simulink model "SchemaControlloDecentralizzatoSmartSixR2013a"  (Simulink 8.7)
settings: Solver=ode45  StartTime=0.0  StopTime=t(end)+Tf  FixedStep=T  MaxStep=T  RelTol=1e-3
PreLoadFcn:
  | initFunction
InitFcn:
  | initFunction
StopFcn:
  | cd ..
  | 
  | figure
  | subplot(31,1)
  | plot(err_q.data(1:50))
  | subplot(312)
  | plot(err_dq.data(1:50))
  | subplot(313)
  | plot(err_ddq.data(1:50))
values from neighbouring files (symbols this model uses):
  FM = Kr^-1*Fv*Kr^-1    [initFunction.m]
  Im = Kr^-1*Bconst*Kr^-1    [initFunction.m]
  KCA = [586.881582263 0 0 0 0 0 0 566.981582263 0 0 0 0 ... (36 elements, 6x6)]    [KCA.mat]
  KCP = [63 0 0 0 0 0 0 63 0 0 0 0 ... (36 elements, 6x6)]    [KCP.mat]
  KCV = [315.577034284 0 0 0 0 0 0 325.715347644 0 0 0 0 ... (36 elements, 6x6)]    [KCV.mat]    (also in initFunction.m = KCV*rKCV^-1)
  KM = [0.0232558139535 0 0 0 0 0 0 0.0158982511924 0 0 0 0 ... (36 elements, 6x6)]    [KM.mat]
  Kr = diag(kr)    [ParametriMotori.m]
  Kt = diag(kt)    [ParametriMotori.m]
  KTA = [1 0 0 0 0 0 0 1 0 0 0 0 ... (36 elements, 6x6)]    [KTA.mat]
  KTP = [1 0 0 0 0 0 0 1 0 0 0 0 ... (36 elements, 6x6)]    [KTP.mat]
  KTV = [1 0 0 0 0 0 0 1 0 0 0 0 ... (36 elements, 6x6)]    [KTV.mat]
  Kv = diag(kv)    [ParametriMotori.m]
  La = diag(la)    [ParametriMotori.m]
  q0 = q0'    [initFunction.m]
  Ra = diag(ra)    [ParametriMotori.m]
  T = Tf    (= 0.002)    [initFunction.m]
  TCA = [4.96122857983e-05 0 0 0 0 0 0 3.97711481373e-05 0 0 0 0 ... (36 elements, 6x6)]    [TCA.mat]
libraries: simulink x18
(part 1 of 2)
CloseFcn:
  | rtwprivate ssgencode ModelCloseRequest ContributiCoppieComau
settings Model: Creator=Alessandro  LastModifiedBy=Gianluigi  ExtModeAutoUpdateStatusClock=off
settings DataIOCC: SaveFormat=StructureWithTime
settings OptimizationCC: BlockReduction=off  BufferReuse=off  ExpressionDepthLimit=2147483647  InitFltsAndDblsToZero=on
settings DebuggingCC: AlgebraicLoopMsg=none  SaveWithParameterizedLinksMsg=none  SignalResolutionControl=TryResolveAllWithWarning  InheritedTsInSrcMsg=none  MultiTaskDSMMsg=warning  MultiTaskCondExecSysMsg=none  TasksWithSamePriorityMsg=none  FcnCallInpInsideContextMsg=UseLocalSettings  UnconnectedInputMsg=none  UnconnectedOutputMsg=none  UnconnectedLineMsg=none  StateNameClashWarn=warning
settings GRTTargetCC: TargetFcnLib=ansi_tfl_tmw.mat  CombineOutputUpdateFcns=off  GRTInterface=on

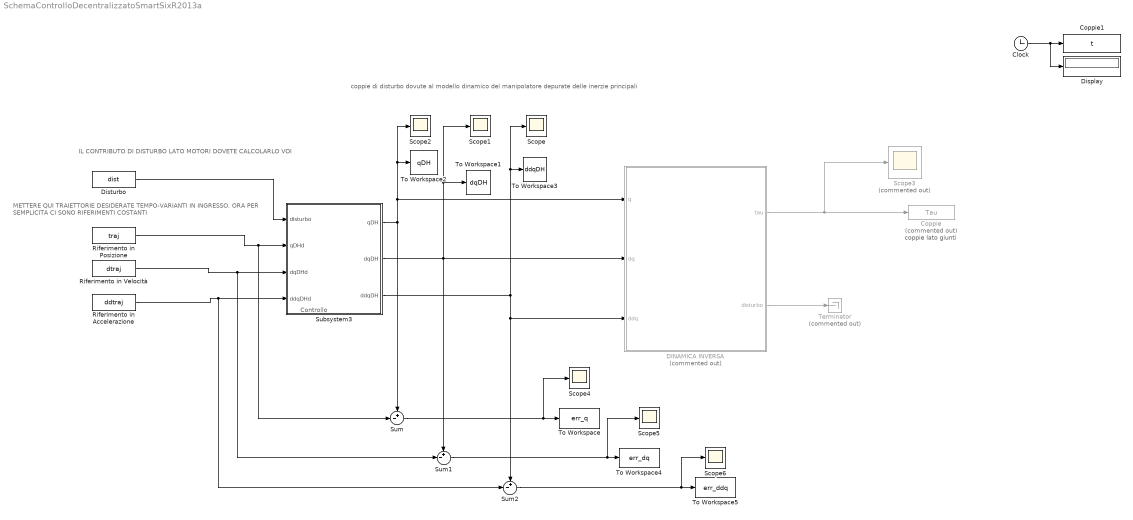
== system SchemaControlloDecentralizzatoSmartSixR2013a ==
  note: coppie di disturbo dovute al modello dinamico del manipolatore depurate delle inerzie principali
  note: Controllo
  note: METTERE QUI TRAIETTORIE DESIDERATE TEMPO-VARIANTI IN INGRESSO.
      | ORA PER SEMPLICITA CI SONO RIFERIMENTI COSTANTI
  note: coppie lato giunti
  note: IL CONTRIBUTO DI DISTURBO LATO MOTORI DOVETE CALCOLARLO VOI
  Clock : Clock
  Coppie : ToWorkspace  Commented=on  VariableName=Tau  SampleTime=-1
  Coppie1 : ToWorkspace  VariableName=t  SampleTime=-1
  DINAMICA INVERSA : Subsystem  Commented=on
      mask Display:
      | disp('Contributi Coppie');
      | port_label('input', 1, 'qDH');
      | port_label('input', 2, 'dqDH');
      | port_label('input', 3, 'ddqDH');
      | port_label('output', 1, 'Coppie Complessive');
      | port_label('output', 2, 'Disturbo lato motori');
  Display : Display
  Disturbo : FromWorkspace  VariableName=dist  Interpolate=off  OutputAfterFinalValue=Holding final value
  Riferimento in Accelerazione : FromWorkspace  VariableName=ddtraj  OutputAfterFinalValue=Holding final value
  Riferimento in Posizione : FromWorkspace  VariableName=traj  Interpolate=off  OutputAfterFinalValue=Holding final value
  Riferimento in Velocità : FromWorkspace  VariableName=dtraj  Interpolate=off  OutputAfterFinalValue=Holding final value
  Scope{,1..2,4..6} (6 alike) : Scope
  Scope3 : Scope  Commented=on
  Subsystem3 : Subsystem
      mask Display:
      | disp('Controllo');
      | port_label('input', 1, 'disturbo');
      | port_label('input', 2, 'qDHd');
      | port_label('input', 3, 'dqDHd');
      | port_label('output', 1, 'qDH');
      | port_label('output', 2, 'dqDH');
      | port_label('output', 3, 'ddqDH');
  Sum : Sum  Inputs=+-|
  Sum1 : Sum  Inputs=+-|
  Sum2 : Sum  Inputs=+-|
  Terminator : Terminator  Commented=on
  To Workspace : ToWorkspace  VariableName=err_q  SaveFormat=Timeseries  SampleTime=-1
  To Workspace1 : ToWorkspace  VariableName=dqDH  SampleTime=-1
  To Workspace2 : ToWorkspace  VariableName=qDH  SampleTime=-1
  To Workspace3 : ToWorkspace  VariableName=ddqDH  SampleTime=-1
  To Workspace4 : ToWorkspace  VariableName=err_dq  SaveFormat=Timeseries  SampleTime=-1
  To Workspace5 : ToWorkspace  VariableName=err_ddq  SaveFormat=Timeseries  SampleTime=-1
  wires:
  Clock/1 -> Coppie1/1, Display/1
  Subsystem3/2(dqDH) -> Sum1/1, To Workspace1/1, Scope1/1, DINAMICA INVERSA/2(dq)
  DINAMICA INVERSA/1(tau) -> Coppie/1, Scope3/1
  Subsystem3/1(qDH) -> DINAMICA INVERSA/1(q), To Workspace2/1, Scope2/1, Sum/1
  Subsystem3/3(ddqDH) -> Sum2/1, DINAMICA INVERSA/3(ddq), To Workspace3/1, Scope/1
  Riferimento in Velocità/1 -> Sum1/2, Subsystem3/3(dqDHd)
  Riferimento in Accelerazione/1 -> Sum2/2, Subsystem3/4(ddqDHd)
  Riferimento in Posizione/1 -> Sum/2, Subsystem3/2(qDHd)
  Disturbo/1 -> Subsystem3/1(disturbo)
  DINAMICA INVERSA/2(disturbo) -> Terminator/1
  Sum/1 -> Scope4/1, To Workspace/1
  Sum1/1 -> Scope5/1, To Workspace4/1
  Sum2/1 -> Scope6/1, To Workspace5/1

== system SchemaControlloDecentralizzatoSmartSixR2013a/DINAMICA INVERSA ==
  note: IL CONTRIBUTO DI DISTURBO LATO MOTORI DOVETE CALCOLARLO VOI
  q : Inport
  dq : Inport  Port=2
  ddq : Inport  Port=3
  Add : Sum  Inputs=++++
  Constant : Constant  Value=[1 1 1 1 1 1]
  Demux : Demux
  Dinamica Inversa : MATLABFcn  MATLABFcn=CalcCoppieComau  OutputDimensions=24
  Mux : Mux  Inputs=3
  To Workspace1 : ToWorkspace  VariableName=tauCentrifugo  SampleTime=-1
  To Workspace2 : ToWorkspace  VariableName=tauAttrViscoso  SampleTime=-1
  To Workspace4 : ToWorkspace  VariableName=tauInerzia  SampleTime=-1
  To Workspace5 : ToWorkspace  VariableName=tauGravita  SampleTime=-1
  tau : Outport
  disturbo : Outport  Port=2
  wires:
  q/1 -> Mux/1
  Mux/1 -> Dinamica Inversa/1
  dq/1 -> Mux/2
  ddq/1 -> Mux/3
  Dinamica Inversa/1 -> Demux/1
  Add/1 -> tau/1
  Demux/1 -> Add/1, To Workspace4/1
  Demux/2 -> Add/2, To Workspace1/1
  Demux/3 -> Add/3, To Workspace2/1
  Demux/4 -> Add/4, To Workspace5/1
  Constant/1 -> disturbo/1

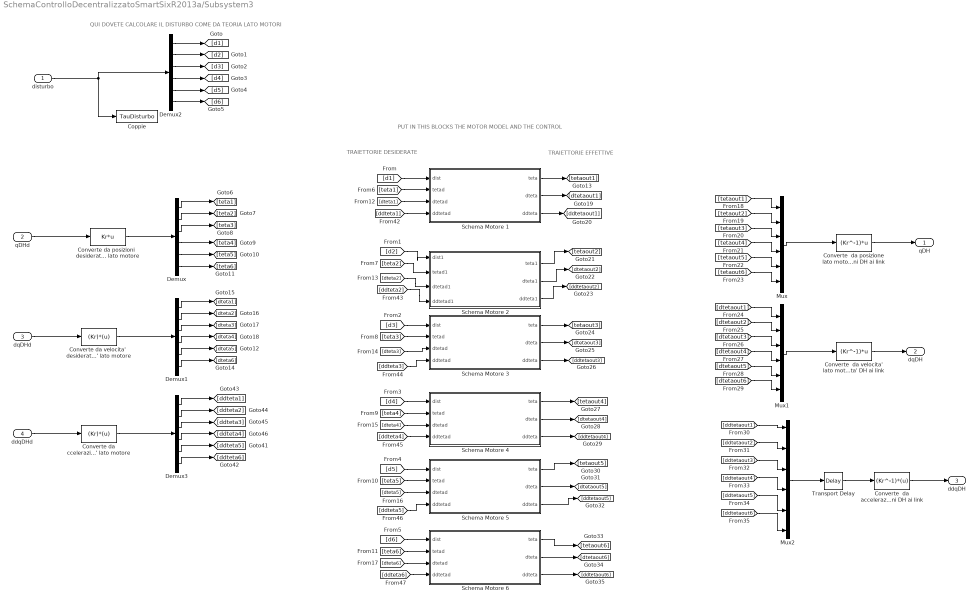
== system SchemaControlloDecentralizzatoSmartSixR2013a/Subsystem3 ==
  note: PUT IN THIS BLOCKS THE MOTOR MODEL AND THE CONTROL
  note: TRAIETTORIE DESIDERATE
  note: TRAIETTORIE EFFETTIVE
  note: QUI DOVETE CALCOLARE IL DISTURBO COME DA TEORIA LATO MOTORI
  disturbo : Inport
  qDHd : Inport  Port=2
  dqDHd : Inport  Port=3
  ddqDHd : Inport  Port=4
  Converte  da accelerazioni lato motore  ad accelerazioni DH ai link : MATLABFcn  MATLABFcn=(Kr^-1)*(u)
  "Converte  da posizione lato motore a  posizioni DH ai link " : MATLABFcn  MATLABFcn=(Kr^-1)*u
  "Converte  da velocita' lato motore  a velocita' DH ai link " : MATLABFcn  MATLABFcn=(Kr^-1)*u
  Converte da ccelerazioni  desiderate DH ai link  in velocita' lato motore : MATLABFcn  MATLABFcn=(Kr)*(u)
  "Converte da posizioni  desiderate DH ai link  in posizione lato motore " : MATLABFcn  MATLABFcn=Kr*u
  "Converte da velocita'  desiderate DH ai link  in velocita' lato motore " : MATLABFcn  MATLABFcn=(Kr)*(u)
  Coppie : ToWorkspace  VariableName=TauDisturbo  SampleTime=-1
  Demux{,1..3} (4 alike) : Demux  Outputs=6
  Mux : Mux  Inputs=6
  Mux1 : Mux  Inputs=6
  Mux2 : Mux  Inputs=6
  Schema Motore 1 : Subsystem  mask{i=1}
  Schema Motore 2 : Subsystem  mask{i=2}
  Schema Motore 3 : Subsystem  mask{i=3}
  Schema Motore 4 : Subsystem  mask{i=4}
  Schema Motore 5 : Subsystem  mask{i=5}
  Schema Motore 6 : Subsystem  mask{i=6}
  Transport Delay : TransportDelay  DelayTime=T
  qDH : Outport
  dqDH : Outport  Port=2
  ddqDH : Outport  Port=3
  wires:
  qDHd/1 -> "Converte da posizioni  desiderate DH ai link  in posizione lato motore "/1
  dqDHd/1 -> "Converte da velocita'  desiderate DH ai link  in velocita' lato motore "/1
  "Converte  da velocita' lato motore  a velocita' DH ai link "/1 -> dqDH/1
  Converte  da accelerazioni lato motore  ad accelerazioni DH ai link/1 -> ddqDH/1
  "Converte da posizioni  desiderate DH ai link  in posizione lato motore "/1 -> Demux/1
  disturbo/1 -> Coppie/1, Demux2/1
  "Converte  da posizione lato motore a  posizioni DH ai link "/1 -> qDH/1
  Mux/1 -> "Converte  da posizione lato motore a  posizioni DH ai link "/1
  Demux2/1 -> [d1]
  Demux2/2 -> [d2]
  Demux2/3 -> [d3]
  Demux2/4 -> [d4]
  Demux2/5 -> [d5]
  Demux2/6 -> [d6]
  [d3] -> Schema Motore 3/1(dist)
  [d4] -> Schema Motore 4/1(dist)
  [d5] -> Schema Motore 5/1(dist)
  [d6] -> Schema Motore 6/1(dist)
  Demux/1 -> [teta1]
  Demux/2 -> [teta2]
  Demux/3 -> [teta3]
  Demux/4 -> [teta4]
  Demux/5 -> [teta5]
  Demux/6 -> [teta6]
  [teta3] -> Schema Motore 3/2(tetad)
  [teta4] -> Schema Motore 4/2(tetad)
  [teta5] -> Schema Motore 5/2(tetad)
  [teta6] -> Schema Motore 6/2(tetad)
  "Converte da velocita'  desiderate DH ai link  in velocita' lato motore "/1 -> Demux1/1
  Demux1/1 -> [dteta1]
  Demux1/2 -> [dteta2]
  Demux1/3 -> [dteta3]
  Demux1/4 -> [dteta4]
  Demux1/5 -> [dteta5]
  Demux1/6 -> [dteta6]
  [dteta3] -> Schema Motore 3/3(dtetad)
  [dteta4] -> Schema Motore 4/3(dtetad)
  [dteta5] -> Schema Motore 5/3(dtetad)
  [dteta6] -> Schema Motore 6/3(dtetad)
  [tetaout1] -> Mux/1
  [tetaout2] -> Mux/2
  [tetaout3] -> Mux/3
  [tetaout4] -> Mux/4
  [tetaout5] -> Mux/5
  [tetaout6] -> Mux/6
  Mux1/1 -> "Converte  da velocita' lato motore  a velocita' DH ai link "/1
  [dtetaout1] -> Mux1/1
  [dtetaout2] -> Mux1/2
  [dtetaout3] -> Mux1/3
  [dtetaout4] -> Mux1/4
  [dtetaout5] -> Mux1/5
  [dtetaout6] -> Mux1/6
  [ddtetaout1] -> Mux2/1
  [ddtetaout2] -> Mux2/2
  [ddtetaout3] -> Mux2/3
  [ddtetaout4] -> Mux2/4
  [ddtetaout5] -> Mux2/5
  [ddtetaout6] -> Mux2/6
  [teta1] -> Schema Motore 1/2(tetad)
  [dteta1] -> Schema Motore 1/3(dtetad)
  Schema Motore 1/1(teta) -> [tetaout1]
  Schema Motore 1/2(dteta) -> [dtetaout1]
  Schema Motore 1/3(ddteta) -> [ddtetaout1]
  [d1] -> Schema Motore 1/1(dist)
  ddqDHd/1 -> Converte da ccelerazioni  desiderate DH ai link  in velocita' lato motore/1
  Demux3/1 -> [ddteta1]
  Demux3/2 -> [ddteta2]
  Demux3/3 -> [ddteta3]
  Demux3/4 -> [ddteta4]
  Demux3/5 -> [ddteta5]
  Demux3/6 -> [ddteta6]
  Converte da ccelerazioni  desiderate DH ai link  in velocita' lato motore/1 -> Demux3/1
  [ddteta1] -> Schema Motore 1/4(ddtetad)
  Schema Motore 3/1(teta) -> [tetaout3]
  Schema Motore 3/2(dteta) -> [dtetaout3]
  Schema Motore 3/3(ddteta) -> [ddtetaout3]
  Schema Motore 4/1(teta) -> [tetaout4]
  Schema Motore 4/2(dteta) -> [dtetaout4]
  Schema Motore 4/3(ddteta) -> [ddtetaout4]
  Schema Motore 5/1(teta) -> [tetaout5]
  Schema Motore 5/2(dteta) -> [dtetaout5]
  Schema Motore 5/3(ddteta) -> [ddtetaout5]
  Schema Motore 6/1(teta) -> [tetaout6]
  Schema Motore 6/2(dteta) -> [dtetaout6]
  Schema Motore 6/3(ddteta) -> [ddtetaout6]
  [ddteta3] -> Schema Motore 3/4(ddtetad)
  [ddteta4] -> Schema Motore 4/4(ddtetad)
  [ddteta5] -> Schema Motore 5/4(ddtetad)
  [ddteta6] -> Schema Motore 6/4(ddtetad)
  [d2] -> Schema Motore 2/1(dist1)
  [teta2] -> Schema Motore 2/2(tetad1)
  [dteta2] -> Schema Motore 2/3(dtetad1)
  [ddteta2] -> Schema Motore 2/4(ddtetad1)
  Schema Motore 2/1(teta1) -> [tetaout2]
  Schema Motore 2/2(dteta1) -> [dtetaout2]
  Schema Motore 2/3(ddteta1) -> [ddtetaout2]
  Mux2/1 -> Transport Delay/1
  Transport Delay/1 -> Converte  da accelerazioni lato motore  ad accelerazioni DH ai link/1

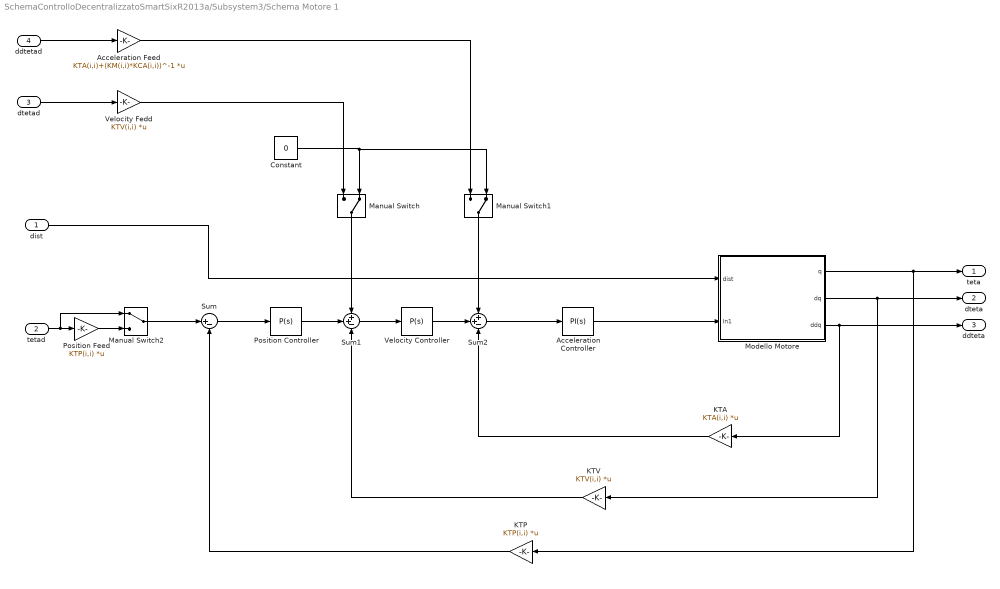
== system SchemaControlloDecentralizzatoSmartSixR2013a/Subsystem3/Schema Motore 1 ==
  dist : Inport  PortDimensions=1
  tetad : Inport  Port=2  PortDimensions=1
  dtetad : Inport  Port=3  PortDimensions=1
  ddtetad : Inport  Port=4  PortDimensions=1
  Acceleration Controller : simulink/Continuous/PID Controller  Controller=PI  TimeDomain=Continuous-time  SampleTime=-1  IntegratorMethod=Forward Euler  FilterMethod=Forward Euler  Form=Parallel  UseFilter=on  ControllerParametersSource=internal  P=TCA(i,i)*KCA(i,i)  I=KCA(i,i)  D=0  N=100  InitialConditionSource=internal  InitialConditionForIntegrator=0  InitialConditionForFilter=0  ExternalReset=none  LimitOutput=off  UpperSaturationLimit=inf  LowerSaturationLimit=-inf  LinearizeAsGain=on  AntiWindupMode=none  Kb=1  TrackingMode=off  Kt=1  PParamMin=[]  PParamMax=[]  IParamMin=[]  IParamMax=[]  DParamMin=[]  DParamMax=[]  NParamMin=[]  NParamMax=[]  KbParamMin=[]  KbParamMax=[]  KtParamMin=[]  KtParamMax=[]  POutMin=[]  POutMax=[]  IOutMin=[]  IOutMax=[]  DOutMin=[]  DOutMax=[]  NOutMin=[]  NOutMax=[]  KbOutMin=[]  KbOutMax=[]  KtOutMin=[]  KtOutMax=[]  IntegratorOutMin=[]  IntegratorOutMax=[]  FilterOutMin=[]  FilterOutMax=[]  SumOutMin=[]  SumOutMax=[]  SumI1OutMin=[]  SumI1OutMax=[]  SumI2OutMin=[]  SumI2OutMax=[]  SumI3OutMin=[]  SumI3OutMax=[]  SumDOutMin=[]  SumDOutMax=[]  SaturationOutMin=[]  SaturationOutMax=[]  IntegratorContinuousStateAttributes=''  IntegratorStateMustResolveToSignalObject=off  IntegratorRTWStateStorageClass=Auto  FilterContinuousStateAttributes=''  FilterStateMustResolveToSignalObject=off  FilterRTWStateStorageClass=Auto  DifferentiatorICPrevScaledInput=0  DifferentiatorOutMin=[]  DifferentiatorOutMax=[]
  Acceleration Feed : Gain  Gain=KTA(i,i)+(KM(i,i)*KCA(i,i))^-1  Multiplication=Matrix(K*u)
  Constant : Constant  Value=0
  KTA : Gain  Gain=KTA(i,i)  Multiplication=Matrix(K*u)
  KTP : Gain  Gain=KTP(i,i)  Multiplication=Matrix(K*u)
  KTV : Gain  Gain=KTV(i,i)  Multiplication=Matrix(K*u)
  Manual Switch : ManualSwitch  CurrentSetting=0
  Manual Switch1 : ManualSwitch  CurrentSetting=0
  Manual Switch2 : ManualSwitch
  Modello Motore : Subsystem
  Position Controller : simulink/Continuous/PID Controller  Controller=P  TimeDomain=Continuous-time  SampleTime=-1  IntegratorMethod=Forward Euler  FilterMethod=Forward Euler  Form=Parallel  UseFilter=on  ControllerParametersSource=internal  P=KCP(i,i)  I=1  D=0  N=100  InitialConditionSource=internal  InitialConditionForIntegrator=0  InitialConditionForFilter=0  ExternalReset=none  LimitOutput=off  UpperSaturationLimit=inf  LowerSaturationLimit=-inf  LinearizeAsGain=on  AntiWindupMode=none  Kb=1  TrackingMode=off  Kt=1  PParamMin=[]  PParamMax=[]  IParamMin=[]  IParamMax=[]  DParamMin=[]  DParamMax=[]  NParamMin=[]  NParamMax=[]  KbParamMin=[]  KbParamMax=[]  KtParamMin=[]  KtParamMax=[]  POutMin=[]  POutMax=[]  IOutMin=[]  IOutMax=[]  DOutMin=[]  DOutMax=[]  NOutMin=[]  NOutMax=[]  KbOutMin=[]  KbOutMax=[]  KtOutMin=[]  KtOutMax=[]  IntegratorOutMin=[]  IntegratorOutMax=[]  FilterOutMin=[]  FilterOutMax=[]  SumOutMin=[]  SumOutMax=[]  SumI1OutMin=[]  SumI1OutMax=[]  SumI2OutMin=[]  SumI2OutMax=[]  SumI3OutMin=[]  SumI3OutMax=[]  SumDOutMin=[]  SumDOutMax=[]  SaturationOutMin=[]  SaturationOutMax=[]  IntegratorContinuousStateAttributes=''  IntegratorStateMustResolveToSignalObject=off  IntegratorRTWStateStorageClass=Auto  FilterContinuousStateAttributes=''  FilterStateMustResolveToSignalObject=off  FilterRTWStateStorageClass=Auto  DifferentiatorICPrevScaledInput=0  DifferentiatorOutMin=[]  DifferentiatorOutMax=[]
  Position Feed : Gain  Gain=KTP(i,i)  Multiplication=Matrix(K*u)
  Sum : Sum  Inputs=|+-
  Sum1 : Sum  Inputs=++-
  Sum2 : Sum  Inputs=++-
  Velocity Controller : simulink/Continuous/PID Controller  Controller=P  TimeDomain=Continuous-time  SampleTime=-1  IntegratorMethod=Forward Euler  FilterMethod=Forward Euler  Form=Parallel  UseFilter=on  ControllerParametersSource=internal  P=KCV(i,i)  I=1  D=0  N=100  InitialConditionSource=internal  InitialConditionForIntegrator=0  InitialConditionForFilter=0  ExternalReset=none  LimitOutput=off  UpperSaturationLimit=inf  LowerSaturationLimit=-inf  LinearizeAsGain=on  AntiWindupMode=none  Kb=1  TrackingMode=off  Kt=1  PParamMin=[]  PParamMax=[]  IParamMin=[]  IParamMax=[]  DParamMin=[]  DParamMax=[]  NParamMin=[]  NParamMax=[]  KbParamMin=[]  KbParamMax=[]  KtParamMin=[]  KtParamMax=[]  POutMin=[]  POutMax=[]  IOutMin=[]  IOutMax=[]  DOutMin=[]  DOutMax=[]  NOutMin=[]  NOutMax=[]  KbOutMin=[]  KbOutMax=[]  KtOutMin=[]  KtOutMax=[]  IntegratorOutMin=[]  IntegratorOutMax=[]  FilterOutMin=[]  FilterOutMax=[]  SumOutMin=[]  SumOutMax=[]  SumI1OutMin=[]  SumI1OutMax=[]  SumI2OutMin=[]  SumI2OutMax=[]  SumI3OutMin=[]  SumI3OutMax=[]  SumDOutMin=[]  SumDOutMax=[]  SaturationOutMin=[]  SaturationOutMax=[]  IntegratorContinuousStateAttributes=''  IntegratorStateMustResolveToSignalObject=off  IntegratorRTWStateStorageClass=Auto  FilterContinuousStateAttributes=''  FilterStateMustResolveToSignalObject=off  FilterRTWStateStorageClass=Auto  DifferentiatorICPrevScaledInput=0  DifferentiatorOutMin=[]  DifferentiatorOutMax=[]
  Velocity Fedd : Gain  Gain=KTV(i,i)  Multiplication=Matrix(K*u)
  teta : Outport  PortDimensions=1
  dteta : Outport  Port=2  PortDimensions=1
  ddteta : Outport  Port=3  PortDimensions=1
  wires:
  Sum/1 -> Position Controller/1
  Sum1/1 -> Velocity Controller/1
  Sum2/1 -> Acceleration Controller/1
  ddtetad/1 -> Acceleration Feed/1
  KTP/1 -> Sum/2
  Acceleration Controller/1 -> Modello Motore/2(In1)
  dist/1 -> Modello Motore/1(dist)
  Modello Motore/2(dq) -> KTV/1, dteta/1
  Modello Motore/1(q) -> KTP/1, teta/1
  Modello Motore/3(ddq) -> KTA/1, ddteta/1
  Position Controller/1 -> Sum1/2
  KTV/1 -> Sum1/3
  Manual Switch/1 -> Sum1/1
  KTA/1 -> Sum2/3
  Velocity Controller/1 -> Sum2/2
  dtetad/1 -> Velocity Fedd/1
  Constant/1 -> Manual Switch1/2, Manual Switch/2
  Manual Switch1/1 -> Sum2/1
  tetad/1 -> Manual Switch2/1, Position Feed/1
  Manual Switch2/1 -> Sum/1
  Position Feed/1 -> Manual Switch2/2
  Velocity Fedd/1 -> Manual Switch/1
  Acceleration Feed/1 -> Manual Switch1/1

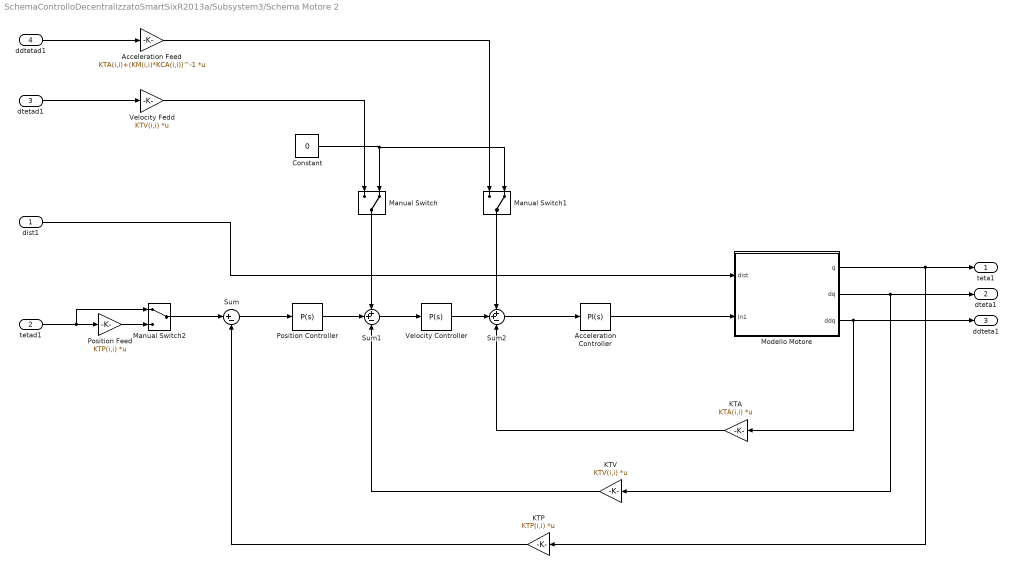
== system SchemaControlloDecentralizzatoSmartSixR2013a/Subsystem3/Schema Motore 2 ==
  dist1 : Inport  PortDimensions=1
  tetad1 : Inport  Port=2  PortDimensions=1
  dtetad1 : Inport  Port=3  PortDimensions=1
  ddtetad1 : Inport  Port=4  PortDimensions=1
  Acceleration Controller : simulink/Continuous/PID Controller  Controller=PI  TimeDomain=Continuous-time  SampleTime=-1  IntegratorMethod=Forward Euler  FilterMethod=Forward Euler  Form=Parallel  UseFilter=on  ControllerParametersSource=internal  P=TCA(i,i)*KCA(i,i)  I=KCA(i,i)  D=0  N=100  InitialConditionSource=internal  InitialConditionForIntegrator=0  InitialConditionForFilter=0  ExternalReset=none  LimitOutput=off  UpperSaturationLimit=inf  LowerSaturationLimit=-inf  LinearizeAsGain=on  AntiWindupMode=none  Kb=1  TrackingMode=off  Kt=1  PParamMin=[]  PParamMax=[]  IParamMin=[]  IParamMax=[]  DParamMin=[]  DParamMax=[]  NParamMin=[]  NParamMax=[]  KbParamMin=[]  KbParamMax=[]  KtParamMin=[]  KtParamMax=[]  POutMin=[]  POutMax=[]  IOutMin=[]  IOutMax=[]  DOutMin=[]  DOutMax=[]  NOutMin=[]  NOutMax=[]  KbOutMin=[]  KbOutMax=[]  KtOutMin=[]  KtOutMax=[]  IntegratorOutMin=[]  IntegratorOutMax=[]  FilterOutMin=[]  FilterOutMax=[]  SumOutMin=[]  SumOutMax=[]  SumI1OutMin=[]  SumI1OutMax=[]  SumI2OutMin=[]  SumI2OutMax=[]  SumI3OutMin=[]  SumI3OutMax=[]  SumDOutMin=[]  SumDOutMax=[]  SaturationOutMin=[]  SaturationOutMax=[]  IntegratorContinuousStateAttributes=''  IntegratorStateMustResolveToSignalObject=off  IntegratorRTWStateStorageClass=Auto  FilterContinuousStateAttributes=''  FilterStateMustResolveToSignalObject=off  FilterRTWStateStorageClass=Auto  DifferentiatorICPrevScaledInput=0  DifferentiatorOutMin=[]  DifferentiatorOutMax=[]
  Acceleration Feed : Gain  Gain=KTA(i,i)+(KM(i,i)*KCA(i,i))^-1  Multiplication=Matrix(K*u)
  Constant : Constant  Value=0
  KTA : Gain  Gain=KTA(i,i)  Multiplication=Matrix(K*u)
  KTP : Gain  Gain=KTP(i,i)  Multiplication=Matrix(K*u)
  KTV : Gain  Gain=KTV(i,i)  Multiplication=Matrix(K*u)
  Manual Switch : ManualSwitch  CurrentSetting=0
  Manual Switch1 : ManualSwitch  CurrentSetting=0
  Manual Switch2 : ManualSwitch
  Modello Motore : Subsystem
  Position Controller : simulink/Continuous/PID Controller  Controller=P  TimeDomain=Continuous-time  SampleTime=-1  IntegratorMethod=Forward Euler  FilterMethod=Forward Euler  Form=Parallel  UseFilter=on  ControllerParametersSource=internal  P=KCP(i,i)  I=1  D=0  N=100  InitialConditionSource=internal  InitialConditionForIntegrator=0  InitialConditionForFilter=0  ExternalReset=none  LimitOutput=off  UpperSaturationLimit=inf  LowerSaturationLimit=-inf  LinearizeAsGain=on  AntiWindupMode=none  Kb=1  TrackingMode=off  Kt=1  PParamMin=[]  PParamMax=[]  IParamMin=[]  IParamMax=[]  DParamMin=[]  DParamMax=[]  NParamMin=[]  NParamMax=[]  KbParamMin=[]  KbParamMax=[]  KtParamMin=[]  KtParamMax=[]  POutMin=[]  POutMax=[]  IOutMin=[]  IOutMax=[]  DOutMin=[]  DOutMax=[]  NOutMin=[]  NOutMax=[]  KbOutMin=[]  KbOutMax=[]  KtOutMin=[]  KtOutMax=[]  IntegratorOutMin=[]  IntegratorOutMax=[]  FilterOutMin=[]  FilterOutMax=[]  SumOutMin=[]  SumOutMax=[]  SumI1OutMin=[]  SumI1OutMax=[]  SumI2OutMin=[]  SumI2OutMax=[]  SumI3OutMin=[]  SumI3OutMax=[]  SumDOutMin=[]  SumDOutMax=[]  SaturationOutMin=[]  SaturationOutMax=[]  IntegratorContinuousStateAttributes=''  IntegratorStateMustResolveToSignalObject=off  IntegratorRTWStateStorageClass=Auto  FilterContinuousStateAttributes=''  FilterStateMustResolveToSignalObject=off  FilterRTWStateStorageClass=Auto  DifferentiatorICPrevScaledInput=0  DifferentiatorOutMin=[]  DifferentiatorOutMax=[]
  Position Feed : Gain  Gain=KTP(i,i)  Multiplication=Matrix(K*u)
  Sum : Sum  Inputs=|+-
  Sum1 : Sum  Inputs=++-
  Sum2 : Sum  Inputs=++-
  Velocity Controller : simulink/Continuous/PID Controller  Controller=P  TimeDomain=Continuous-time  SampleTime=-1  IntegratorMethod=Forward Euler  FilterMethod=Forward Euler  Form=Parallel  UseFilter=on  ControllerParametersSource=internal  P=KCV(i,i)  I=1  D=0  N=100  InitialConditionSource=internal  InitialConditionForIntegrator=0  InitialConditionForFilter=0  ExternalReset=none  LimitOutput=off  UpperSaturationLimit=inf  LowerSaturationLimit=-inf  LinearizeAsGain=on  AntiWindupMode=none  Kb=1  TrackingMode=off  Kt=1  PParamMin=[]  PParamMax=[]  IParamMin=[]  IParamMax=[]  DParamMin=[]  DParamMax=[]  NParamMin=[]  NParamMax=[]  KbParamMin=[]  KbParamMax=[]  KtParamMin=[]  KtParamMax=[]  POutMin=[]  POutMax=[]  IOutMin=[]  IOutMax=[]  DOutMin=[]  DOutMax=[]  NOutMin=[]  NOutMax=[]  KbOutMin=[]  KbOutMax=[]  KtOutMin=[]  KtOutMax=[]  IntegratorOutMin=[]  IntegratorOutMax=[]  FilterOutMin=[]  FilterOutMax=[]  SumOutMin=[]  SumOutMax=[]  SumI1OutMin=[]  SumI1OutMax=[]  SumI2OutMin=[]  SumI2OutMax=[]  SumI3OutMin=[]  SumI3OutMax=[]  SumDOutMin=[]  SumDOutMax=[]  SaturationOutMin=[]  SaturationOutMax=[]  IntegratorContinuousStateAttributes=''  IntegratorStateMustResolveToSignalObject=off  IntegratorRTWStateStorageClass=Auto  FilterContinuousStateAttributes=''  FilterStateMustResolveToSignalObject=off  FilterRTWStateStorageClass=Auto  DifferentiatorICPrevScaledInput=0  DifferentiatorOutMin=[]  DifferentiatorOutMax=[]
  Velocity Fedd : Gain  Gain=KTV(i,i)  Multiplication=Matrix(K*u)
  teta1 : Outport  PortDimensions=1
  dteta1 : Outport  Port=2  PortDimensions=1
  ddteta1 : Outport  Port=3  PortDimensions=1
  wires:
  Sum/1 -> Position Controller/1
  Sum1/1 -> Velocity Controller/1
  Sum2/1 -> Acceleration Controller/1
  ddtetad1/1 -> Acceleration Feed/1
  KTP/1 -> Sum/2
  Acceleration Controller/1 -> Modello Motore/2(In1)
  dist1/1 -> Modello Motore/1(dist)
  Modello Motore/2(dq) -> dteta1/1, KTV/1
  Modello Motore/1(q) -> KTP/1, teta1/1
  Modello Motore/3(ddq) -> ddteta1/1, KTA/1
  Position Controller/1 -> Sum1/2
  KTV/1 -> Sum1/3
  Manual Switch/1 -> Sum1/1
  KTA/1 -> Sum2/3
  Velocity Controller/1 -> Sum2/2
  dtetad1/1 -> Velocity Fedd/1
  Constant/1 -> Manual Switch1/2, Manual Switch/2
  Manual Switch1/1 -> Sum2/1
  tetad1/1 -> Position Feed/1, Manual Switch2/1
  Manual Switch2/1 -> Sum/1
  Position Feed/1 -> Manual Switch2/2
  Velocity Fedd/1 -> Manual Switch/1
  Acceleration Feed/1 -> Manual Switch1/1

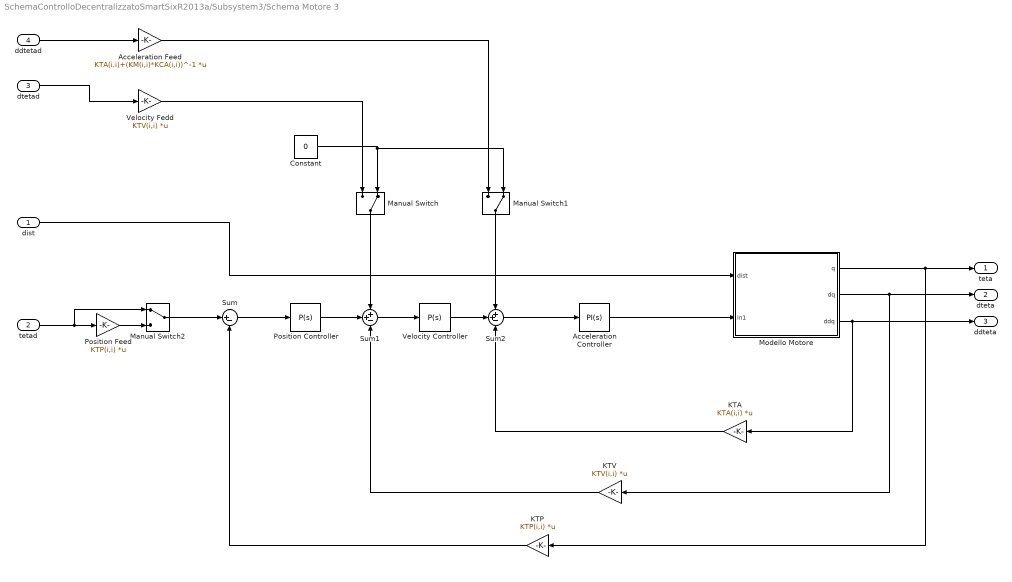
== system SchemaControlloDecentralizzatoSmartSixR2013a/Subsystem3/Schema Motore 3 ==
  dist : Inport  PortDimensions=1
  tetad : Inport  Port=2  PortDimensions=1
  dtetad : Inport  Port=3  PortDimensions=1
  ddtetad : Inport  Port=4  PortDimensions=1
  Acceleration Controller : simulink/Continuous/PID Controller  Controller=PI  TimeDomain=Continuous-time  SampleTime=-1  IntegratorMethod=Forward Euler  FilterMethod=Forward Euler  Form=Parallel  UseFilter=on  ControllerParametersSource=internal  P=TCA(i,i)*KCA(i,i)  I=KCA(i,i)  D=0  N=100  InitialConditionSource=internal  InitialConditionForIntegrator=0  InitialConditionForFilter=0  ExternalReset=none  LimitOutput=off  UpperSaturationLimit=inf  LowerSaturationLimit=-inf  LinearizeAsGain=on  AntiWindupMode=none  Kb=1  TrackingMode=off  Kt=1  PParamMin=[]  PParamMax=[]  IParamMin=[]  IParamMax=[]  DParamMin=[]  DParamMax=[]  NParamMin=[]  NParamMax=[]  KbParamMin=[]  KbParamMax=[]  KtParamMin=[]  KtParamMax=[]  POutMin=[]  POutMax=[]  IOutMin=[]  IOutMax=[]  DOutMin=[]  DOutMax=[]  NOutMin=[]  NOutMax=[]  KbOutMin=[]  KbOutMax=[]  KtOutMin=[]  KtOutMax=[]  IntegratorOutMin=[]  IntegratorOutMax=[]  FilterOutMin=[]  FilterOutMax=[]  SumOutMin=[]  SumOutMax=[]  SumI1OutMin=[]  SumI1OutMax=[]  SumI2OutMin=[]  SumI2OutMax=[]  SumI3OutMin=[]  SumI3OutMax=[]  SumDOutMin=[]  SumDOutMax=[]  SaturationOutMin=[]  SaturationOutMax=[]  IntegratorContinuousStateAttributes=''  IntegratorStateMustResolveToSignalObject=off  IntegratorRTWStateStorageClass=Auto  FilterContinuousStateAttributes=''  FilterStateMustResolveToSignalObject=off  FilterRTWStateStorageClass=Auto  DifferentiatorICPrevScaledInput=0  DifferentiatorOutMin=[]  DifferentiatorOutMax=[]
  Acceleration Feed : Gain  Gain=KTA(i,i)+(KM(i,i)*KCA(i,i))^-1  Multiplication=Matrix(K*u)
  Constant : Constant  Value=0
  KTA : Gain  Gain=KTA(i,i)  Multiplication=Matrix(K*u)
  KTP : Gain  Gain=KTP(i,i)  Multiplication=Matrix(K*u)
  KTV : Gain  Gain=KTV(i,i)  Multiplication=Matrix(K*u)
  Manual Switch : ManualSwitch  CurrentSetting=0
  Manual Switch1 : ManualSwitch  CurrentSetting=0
  Manual Switch2 : ManualSwitch
  Modello Motore : Subsystem
  Position Controller : simulink/Continuous/PID Controller  Controller=P  TimeDomain=Continuous-time  SampleTime=-1  IntegratorMethod=Forward Euler  FilterMethod=Forward Euler  Form=Parallel  UseFilter=on  ControllerParametersSource=internal  P=KCP(i,i)  I=1  D=0  N=100  InitialConditionSource=internal  InitialConditionForIntegrator=0  InitialConditionForFilter=0  ExternalReset=none  LimitOutput=off  UpperSaturationLimit=inf  LowerSaturationLimit=-inf  LinearizeAsGain=on  AntiWindupMode=none  Kb=1  TrackingMode=off  Kt=1  PParamMin=[]  PParamMax=[]  IParamMin=[]  IParamMax=[]  DParamMin=[]  DParamMax=[]  NParamMin=[]  NParamMax=[]  KbParamMin=[]  KbParamMax=[]  KtParamMin=[]  KtParamMax=[]  POutMin=[]  POutMax=[]  IOutMin=[]  IOutMax=[]  DOutMin=[]  DOutMax=[]  NOutMin=[]  NOutMax=[]  KbOutMin=[]  KbOutMax=[]  KtOutMin=[]  KtOutMax=[]  IntegratorOutMin=[]  IntegratorOutMax=[]  FilterOutMin=[]  FilterOutMax=[]  SumOutMin=[]  SumOutMax=[]  SumI1OutMin=[]  SumI1OutMax=[]  SumI2OutMin=[]  SumI2OutMax=[]  SumI3OutMin=[]  SumI3OutMax=[]  SumDOutMin=[]  SumDOutMax=[]  SaturationOutMin=[]  SaturationOutMax=[]  IntegratorContinuousStateAttributes=''  IntegratorStateMustResolveToSignalObject=off  IntegratorRTWStateStorageClass=Auto  FilterContinuousStateAttributes=''  FilterStateMustResolveToSignalObject=off  FilterRTWStateStorageClass=Auto  DifferentiatorICPrevScaledInput=0  DifferentiatorOutMin=[]  DifferentiatorOutMax=[]
  Position Feed : Gain  Gain=KTP(i,i)  Multiplication=Matrix(K*u)
  Sum : Sum  Inputs=|+-
  Sum1 : Sum  Inputs=++-
  Sum2 : Sum  Inputs=++-
  Velocity Controller : simulink/Continuous/PID Controller  Controller=P  TimeDomain=Continuous-time  SampleTime=-1  IntegratorMethod=Forward Euler  FilterMethod=Forward Euler  Form=Parallel  UseFilter=on  ControllerParametersSource=internal  P=KCV(i,i)  I=1  D=0  N=100  InitialConditionSource=internal  InitialConditionForIntegrator=0  InitialConditionForFilter=0  ExternalReset=none  LimitOutput=off  UpperSaturationLimit=inf  LowerSaturationLimit=-inf  LinearizeAsGain=on  AntiWindupMode=none  Kb=1  TrackingMode=off  Kt=1  PParamMin=[]  PParamMax=[]  IParamMin=[]  IParamMax=[]  DParamMin=[]  DParamMax=[]  NParamMin=[]  NParamMax=[]  KbParamMin=[]  KbParamMax=[]  KtParamMin=[]  KtParamMax=[]  POutMin=[]  POutMax=[]  IOutMin=[]  IOutMax=[]  DOutMin=[]  DOutMax=[]  NOutMin=[]  NOutMax=[]  KbOutMin=[]  KbOutMax=[]  KtOutMin=[]  KtOutMax=[]  IntegratorOutMin=[]  IntegratorOutMax=[]  FilterOutMin=[]  FilterOutMax=[]  SumOutMin=[]  SumOutMax=[]  SumI1OutMin=[]  SumI1OutMax=[]  SumI2OutMin=[]  SumI2OutMax=[]  SumI3OutMin=[]  SumI3OutMax=[]  SumDOutMin=[]  SumDOutMax=[]  SaturationOutMin=[]  SaturationOutMax=[]  IntegratorContinuousStateAttributes=''  IntegratorStateMustResolveToSignalObject=off  IntegratorRTWStateStorageClass=Auto  FilterContinuousStateAttributes=''  FilterStateMustResolveToSignalObject=off  FilterRTWStateStorageClass=Auto  DifferentiatorICPrevScaledInput=0  DifferentiatorOutMin=[]  DifferentiatorOutMax=[]
  Velocity Fedd : Gain  Gain=KTV(i,i)  Multiplication=Matrix(K*u)
  teta : Outport  PortDimensions=1
  dteta : Outport  Port=2  PortDimensions=1
  ddteta : Outport  Port=3  PortDimensions=1
  wires:
  Sum/1 -> Position Controller/1
  Sum1/1 -> Velocity Controller/1
  Sum2/1 -> Acceleration Controller/1
  ddtetad/1 -> Acceleration Feed/1
  KTP/1 -> Sum/2
  Acceleration Controller/1 -> Modello Motore/2(In1)
  dist/1 -> Modello Motore/1(dist)
  Modello Motore/2(dq) -> dteta/1, KTV/1
  Modello Motore/1(q) -> teta/1, KTP/1
  Modello Motore/3(ddq) -> ddteta/1, KTA/1
  Position Controller/1 -> Sum1/2
  KTV/1 -> Sum1/3
  Manual Switch/1 -> Sum1/1
  KTA/1 -> Sum2/3
  Velocity Controller/1 -> Sum2/2
  Constant/1 -> Manual Switch1/2, Manual Switch/2
  Manual Switch1/1 -> Sum2/1
  tetad/1 -> Position Feed/1, Manual Switch2/1
  Manual Switch2/1 -> Sum/1
  Position Feed/1 -> Manual Switch2/2
  Velocity Fedd/1 -> Manual Switch/1
  Acceleration Feed/1 -> Manual Switch1/1
  dtetad/1 -> Velocity Fedd/1

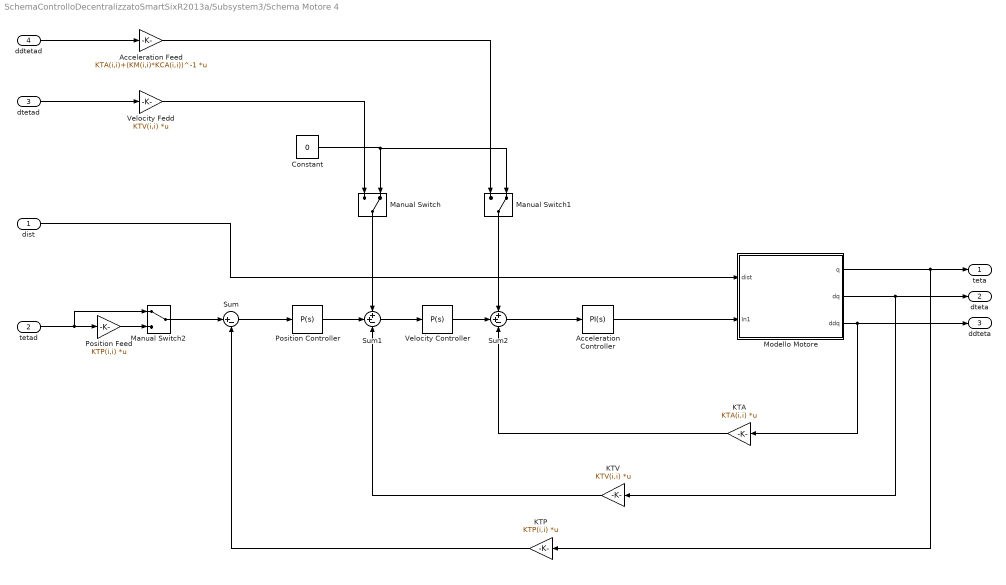
== system SchemaControlloDecentralizzatoSmartSixR2013a/Subsystem3/Schema Motore 4 ==
  dist : Inport  PortDimensions=1
  tetad : Inport  Port=2  PortDimensions=1
  dtetad : Inport  Port=3  PortDimensions=1
  ddtetad : Inport  Port=4  PortDimensions=1
  Acceleration Controller : simulink/Continuous/PID Controller  Controller=PI  TimeDomain=Continuous-time  SampleTime=-1  IntegratorMethod=Forward Euler  FilterMethod=Forward Euler  Form=Parallel  UseFilter=on  ControllerParametersSource=internal  P=TCA(i,i)*KCA(i,i)  I=KCA(i,i)  D=0  N=100  InitialConditionSource=internal  InitialConditionForIntegrator=0  InitialConditionForFilter=0  ExternalReset=none  LimitOutput=off  UpperSaturationLimit=inf  LowerSaturationLimit=-inf  LinearizeAsGain=on  AntiWindupMode=none  Kb=1  TrackingMode=off  Kt=1  PParamMin=[]  PParamMax=[]  IParamMin=[]  IParamMax=[]  DParamMin=[]  DParamMax=[]  NParamMin=[]  NParamMax=[]  KbParamMin=[]  KbParamMax=[]  KtParamMin=[]  KtParamMax=[]  POutMin=[]  POutMax=[]  IOutMin=[]  IOutMax=[]  DOutMin=[]  DOutMax=[]  NOutMin=[]  NOutMax=[]  KbOutMin=[]  KbOutMax=[]  KtOutMin=[]  KtOutMax=[]  IntegratorOutMin=[]  IntegratorOutMax=[]  FilterOutMin=[]  FilterOutMax=[]  SumOutMin=[]  SumOutMax=[]  SumI1OutMin=[]  SumI1OutMax=[]  SumI2OutMin=[]  SumI2OutMax=[]  SumI3OutMin=[]  SumI3OutMax=[]  SumDOutMin=[]  SumDOutMax=[]  SaturationOutMin=[]  SaturationOutMax=[]  IntegratorContinuousStateAttributes=''  IntegratorStateMustResolveToSignalObject=off  IntegratorRTWStateStorageClass=Auto  FilterContinuousStateAttributes=''  FilterStateMustResolveToSignalObject=off  FilterRTWStateStorageClass=Auto  DifferentiatorICPrevScaledInput=0  DifferentiatorOutMin=[]  DifferentiatorOutMax=[]
  Acceleration Feed : Gain  Gain=KTA(i,i)+(KM(i,i)*KCA(i,i))^-1  Multiplication=Matrix(K*u)
  Constant : Constant  Value=0
  KTA : Gain  Gain=KTA(i,i)  Multiplication=Matrix(K*u)
  KTP : Gain  Gain=KTP(i,i)  Multiplication=Matrix(K*u)
  KTV : Gain  Gain=KTV(i,i)  Multiplication=Matrix(K*u)
  Manual Switch : ManualSwitch  CurrentSetting=0
  Manual Switch1 : ManualSwitch  CurrentSetting=0
  Manual Switch2 : ManualSwitch
  Modello Motore : Subsystem
  Position Controller : simulink/Continuous/PID Controller  Controller=P  TimeDomain=Continuous-time  SampleTime=-1  IntegratorMethod=Forward Euler  FilterMethod=Forward Euler  Form=Parallel  UseFilter=on  ControllerParametersSource=internal  P=KCP(i,i)  I=1  D=0  N=100  InitialConditionSource=internal  InitialConditionForIntegrator=0  InitialConditionForFilter=0  ExternalReset=none  LimitOutput=off  UpperSaturationLimit=inf  LowerSaturationLimit=-inf  LinearizeAsGain=on  AntiWindupMode=none  Kb=1  TrackingMode=off  Kt=1  PParamMin=[]  PParamMax=[]  IParamMin=[]  IParamMax=[]  DParamMin=[]  DParamMax=[]  NParamMin=[]  NParamMax=[]  KbParamMin=[]  KbParamMax=[]  KtParamMin=[]  KtParamMax=[]  POutMin=[]  POutMax=[]  IOutMin=[]  IOutMax=[]  DOutMin=[]  DOutMax=[]  NOutMin=[]  NOutMax=[]  KbOutMin=[]  KbOutMax=[]  KtOutMin=[]  KtOutMax=[]  IntegratorOutMin=[]  IntegratorOutMax=[]  FilterOutMin=[]  FilterOutMax=[]  SumOutMin=[]  SumOutMax=[]  SumI1OutMin=[]  SumI1OutMax=[]  SumI2OutMin=[]  SumI2OutMax=[]  SumI3OutMin=[]  SumI3OutMax=[]  SumDOutMin=[]  SumDOutMax=[]  SaturationOutMin=[]  SaturationOutMax=[]  IntegratorContinuousStateAttributes=''  IntegratorStateMustResolveToSignalObject=off  IntegratorRTWStateStorageClass=Auto  FilterContinuousStateAttributes=''  FilterStateMustResolveToSignalObject=off  FilterRTWStateStorageClass=Auto  DifferentiatorICPrevScaledInput=0  DifferentiatorOutMin=[]  DifferentiatorOutMax=[]
  Position Feed : Gain  Gain=KTP(i,i)  Multiplication=Matrix(K*u)
  Sum : Sum  Inputs=|+-
  Sum1 : Sum  Inputs=++-
  Sum2 : Sum  Inputs=++-
  Velocity Controller : simulink/Continuous/PID Controller  Controller=P  TimeDomain=Continuous-time  SampleTime=-1  IntegratorMethod=Forward Euler  FilterMethod=Forward Euler  Form=Parallel  UseFilter=on  ControllerParametersSource=internal  P=KCV(i,i)  I=1  D=0  N=100  InitialConditionSource=internal  InitialConditionForIntegrator=0  InitialConditionForFilter=0  ExternalReset=none  LimitOutput=off  UpperSaturationLimit=inf  LowerSaturationLimit=-inf  LinearizeAsGain=on  AntiWindupMode=none  Kb=1  TrackingMode=off  Kt=1  PParamMin=[]  PParamMax=[]  IParamMin=[]  IParamMax=[]  DParamMin=[]  DParamMax=[]  NParamMin=[]  NParamMax=[]  KbParamMin=[]  KbParamMax=[]  KtParamMin=[]  KtParamMax=[]  POutMin=[]  POutMax=[]  IOutMin=[]  IOutMax=[]  DOutMin=[]  DOutMax=[]  NOutMin=[]  NOutMax=[]  KbOutMin=[]  KbOutMax=[]  KtOutMin=[]  KtOutMax=[]  IntegratorOutMin=[]  IntegratorOutMax=[]  FilterOutMin=[]  FilterOutMax=[]  SumOutMin=[]  SumOutMax=[]  SumI1OutMin=[]  SumI1OutMax=[]  SumI2OutMin=[]  SumI2OutMax=[]  SumI3OutMin=[]  SumI3OutMax=[]  SumDOutMin=[]  SumDOutMax=[]  SaturationOutMin=[]  SaturationOutMax=[]  IntegratorContinuousStateAttributes=''  IntegratorStateMustResolveToSignalObject=off  IntegratorRTWStateStorageClass=Auto  FilterContinuousStateAttributes=''  FilterStateMustResolveToSignalObject=off  FilterRTWStateStorageClass=Auto  DifferentiatorICPrevScaledInput=0  DifferentiatorOutMin=[]  DifferentiatorOutMax=[]
  Velocity Fedd : Gain  Gain=KTV(i,i)  Multiplication=Matrix(K*u)
  teta : Outport  PortDimensions=1
  dteta : Outport  Port=2  PortDimensions=1
  ddteta : Outport  Port=3  PortDimensions=1
  wires:
  Sum/1 -> Position Controller/1
  Sum1/1 -> Velocity Controller/1
  Sum2/1 -> Acceleration Controller/1
  ddtetad/1 -> Acceleration Feed/1
  KTP/1 -> Sum/2
  Acceleration Controller/1 -> Modello Motore/2(In1)
  dist/1 -> Modello Motore/1(dist)
  Modello Motore/2(dq) -> dteta/1, KTV/1
  Modello Motore/1(q) -> teta/1, KTP/1
  Modello Motore/3(ddq) -> ddteta/1, KTA/1
  Position Controller/1 -> Sum1/2
  KTV/1 -> Sum1/3
  Manual Switch/1 -> Sum1/1
  KTA/1 -> Sum2/3
  Velocity Controller/1 -> Sum2/2
  dtetad/1 -> Velocity Fedd/1
  Constant/1 -> Manual Switch1/2, Manual Switch/2
  Manual Switch1/1 -> Sum2/1
  tetad/1 -> Position Feed/1, Manual Switch2/1
  Manual Switch2/1 -> Sum/1
  Position Feed/1 -> Manual Switch2/2
  Velocity Fedd/1 -> Manual Switch/1
  Acceleration Feed/1 -> Manual Switch1/1

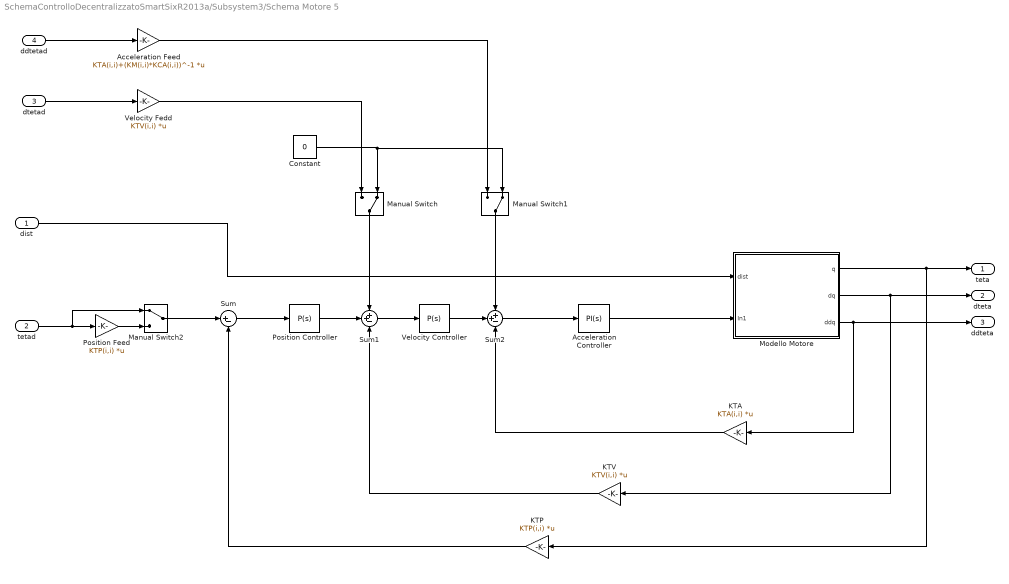
== system SchemaControlloDecentralizzatoSmartSixR2013a/Subsystem3/Schema Motore 5 ==
  dist : Inport  PortDimensions=1
  tetad : Inport  Port=2  PortDimensions=1
  dtetad : Inport  Port=3  PortDimensions=1
  ddtetad : Inport  Port=4  PortDimensions=1
  Acceleration Controller : simulink/Continuous/PID Controller  Controller=PI  TimeDomain=Continuous-time  SampleTime=-1  IntegratorMethod=Forward Euler  FilterMethod=Forward Euler  Form=Parallel  UseFilter=on  ControllerParametersSource=internal  P=TCA(i,i)*KCA(i,i)  I=KCA(i,i)  D=0  N=100  InitialConditionSource=internal  InitialConditionForIntegrator=0  InitialConditionForFilter=0  ExternalReset=none  LimitOutput=off  UpperSaturationLimit=inf  LowerSaturationLimit=-inf  LinearizeAsGain=on  AntiWindupMode=none  Kb=1  TrackingMode=off  Kt=1  PParamMin=[]  PParamMax=[]  IParamMin=[]  IParamMax=[]  DParamMin=[]  DParamMax=[]  NParamMin=[]  NParamMax=[]  KbParamMin=[]  KbParamMax=[]  KtParamMin=[]  KtParamMax=[]  POutMin=[]  POutMax=[]  IOutMin=[]  IOutMax=[]  DOutMin=[]  DOutMax=[]  NOutMin=[]  NOutMax=[]  KbOutMin=[]  KbOutMax=[]  KtOutMin=[]  KtOutMax=[]  IntegratorOutMin=[]  IntegratorOutMax=[]  FilterOutMin=[]  FilterOutMax=[]  SumOutMin=[]  SumOutMax=[]  SumI1OutMin=[]  SumI1OutMax=[]  SumI2OutMin=[]  SumI2OutMax=[]  SumI3OutMin=[]  SumI3OutMax=[]  SumDOutMin=[]  SumDOutMax=[]  SaturationOutMin=[]  SaturationOutMax=[]  IntegratorContinuousStateAttributes=''  IntegratorStateMustResolveToSignalObject=off  IntegratorRTWStateStorageClass=Auto  FilterContinuousStateAttributes=''  FilterStateMustResolveToSignalObject=off  FilterRTWStateStorageClass=Auto  DifferentiatorICPrevScaledInput=0  DifferentiatorOutMin=[]  DifferentiatorOutMax=[]
  Acceleration Feed : Gain  Gain=KTA(i,i)+(KM(i,i)*KCA(i,i))^-1  Multiplication=Matrix(K*u)
  Constant : Constant  Value=0
  KTA : Gain  Gain=KTA(i,i)  Multiplication=Matrix(K*u)
  KTP : Gain  Gain=KTP(i,i)  Multiplication=Matrix(K*u)
  KTV : Gain  Gain=KTV(i,i)  Multiplication=Matrix(K*u)
  Manual Switch : ManualSwitch  CurrentSetting=0
  Manual Switch1 : ManualSwitch  CurrentSetting=0
  Manual Switch2 : ManualSwitch
  Modello Motore : Subsystem
  Position Controller : simulink/Continuous/PID Controller  Controller=P  TimeDomain=Continuous-time  SampleTime=-1  IntegratorMethod=Forward Euler  FilterMethod=Forward Euler  Form=Parallel  UseFilter=on  ControllerParametersSource=internal  P=KCP(i,i)  I=1  D=0  N=100  InitialConditionSource=internal  InitialConditionForIntegrator=0  InitialConditionForFilter=0  ExternalReset=none  LimitOutput=off  UpperSaturationLimit=inf  LowerSaturationLimit=-inf  LinearizeAsGain=on  AntiWindupMode=none  Kb=1  TrackingMode=off  Kt=1  PParamMin=[]  PParamMax=[]  IParamMin=[]  IParamMax=[]  DParamMin=[]  DParamMax=[]  NParamMin=[]  NParamMax=[]  KbParamMin=[]  KbParamMax=[]  KtParamMin=[]  KtParamMax=[]  POutMin=[]  POutMax=[]  IOutMin=[]  IOutMax=[]  DOutMin=[]  DOutMax=[]  NOutMin=[]  NOutMax=[]  KbOutMin=[]  KbOutMax=[]  KtOutMin=[]  KtOutMax=[]  IntegratorOutMin=[]  IntegratorOutMax=[]  FilterOutMin=[]  FilterOutMax=[]  SumOutMin=[]  SumOutMax=[]  SumI1OutMin=[]  SumI1OutMax=[]  SumI2OutMin=[]  SumI2OutMax=[]  SumI3OutMin=[]  SumI3OutMax=[]  SumDOutMin=[]  SumDOutMax=[]  SaturationOutMin=[]  SaturationOutMax=[]  IntegratorContinuousStateAttributes=''  IntegratorStateMustResolveToSignalObject=off  IntegratorRTWStateStorageClass=Auto  FilterContinuousStateAttributes=''  FilterStateMustResolveToSignalObject=off  FilterRTWStateStorageClass=Auto  DifferentiatorICPrevScaledInput=0  DifferentiatorOutMin=[]  DifferentiatorOutMax=[]
  Position Feed : Gain  Gain=KTP(i,i)  Multiplication=Matrix(K*u)
  Sum : Sum  Inputs=|+-
  Sum1 : Sum  Inputs=++-
  Sum2 : Sum  Inputs=++-
  Velocity Controller : simulink/Continuous/PID Controller  Controller=P  TimeDomain=Continuous-time  SampleTime=-1  IntegratorMethod=Forward Euler  FilterMethod=Forward Euler  Form=Parallel  UseFilter=on  ControllerParametersSource=internal  P=KCV(i,i)  I=1  D=0  N=100  InitialConditionSource=internal  InitialConditionForIntegrator=0  InitialConditionForFilter=0  ExternalReset=none  LimitOutput=off  UpperSaturationLimit=inf  LowerSaturationLimit=-inf  LinearizeAsGain=on  AntiWindupMode=none  Kb=1  TrackingMode=off  Kt=1  PParamMin=[]  PParamMax=[]  IParamMin=[]  IParamMax=[]  DParamMin=[]  DParamMax=[]  NParamMin=[]  NParamMax=[]  KbParamMin=[]  KbParamMax=[]  KtParamMin=[]  KtParamMax=[]  POutMin=[]  POutMax=[]  IOutMin=[]  IOutMax=[]  DOutMin=[]  DOutMax=[]  NOutMin=[]  NOutMax=[]  KbOutMin=[]  KbOutMax=[]  KtOutMin=[]  KtOutMax=[]  IntegratorOutMin=[]  IntegratorOutMax=[]  FilterOutMin=[]  FilterOutMax=[]  SumOutMin=[]  SumOutMax=[]  SumI1OutMin=[]  SumI1OutMax=[]  SumI2OutMin=[]  SumI2OutMax=[]  SumI3OutMin=[]  SumI3OutMax=[]  SumDOutMin=[]  SumDOutMax=[]  SaturationOutMin=[]  SaturationOutMax=[]  IntegratorContinuousStateAttributes=''  IntegratorStateMustResolveToSignalObject=off  IntegratorRTWStateStorageClass=Auto  FilterContinuousStateAttributes=''  FilterStateMustResolveToSignalObject=off  FilterRTWStateStorageClass=Auto  DifferentiatorICPrevScaledInput=0  DifferentiatorOutMin=[]  DifferentiatorOutMax=[]
  Velocity Fedd : Gain  Gain=KTV(i,i)  Multiplication=Matrix(K*u)
  teta : Outport  PortDimensions=1
  dteta : Outport  Port=2  PortDimensions=1
  ddteta : Outport  Port=3  PortDimensions=1
  wires:
  Sum/1 -> Position Controller/1
  Sum1/1 -> Velocity Controller/1
  Sum2/1 -> Acceleration Controller/1
  KTP/1 -> Sum/2
  Acceleration Controller/1 -> Modello Motore/2(In1)
  dist/1 -> Modello Motore/1(dist)
  Modello Motore/2(dq) -> dteta/1, KTV/1
  Modello Motore/1(q) -> teta/1, KTP/1
  Modello Motore/3(ddq) -> ddteta/1, KTA/1
  Position Controller/1 -> Sum1/2
  KTV/1 -> Sum1/3
  Manual Switch/1 -> Sum1/1
  KTA/1 -> Sum2/3
  Velocity Controller/1 -> Sum2/2
  Constant/1 -> Manual Switch1/2, Manual Switch/2
  Manual Switch1/1 -> Sum2/1
  tetad/1 -> Position Feed/1, Manual Switch2/1
  Manual Switch2/1 -> Sum/1
  Position Feed/1 -> Manual Switch2/2
  Velocity Fedd/1 -> Manual Switch/1
  Acceleration Feed/1 -> Manual Switch1/1
  dtetad/1 -> Velocity Fedd/1
  ddtetad/1 -> Acceleration Feed/1

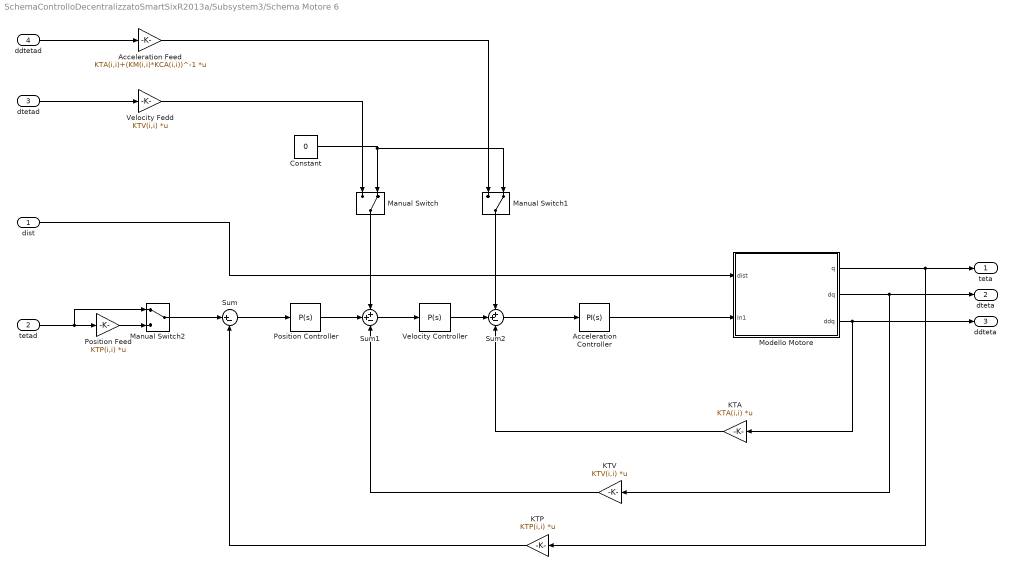
== system SchemaControlloDecentralizzatoSmartSixR2013a/Subsystem3/Schema Motore 6 ==
  dist : Inport  PortDimensions=1
  tetad : Inport  Port=2  PortDimensions=1
  dtetad : Inport  Port=3  PortDimensions=1
  ddtetad : Inport  Port=4  PortDimensions=1
  Acceleration Controller : simulink/Continuous/PID Controller  Controller=PI  TimeDomain=Continuous-time  SampleTime=-1  IntegratorMethod=Forward Euler  FilterMethod=Forward Euler  Form=Parallel  UseFilter=on  ControllerParametersSource=internal  P=TCA(i,i)*KCA(i,i)  I=KCA(i,i)  D=0  N=100  InitialConditionSource=internal  InitialConditionForIntegrator=0  InitialConditionForFilter=0  ExternalReset=none  LimitOutput=off  UpperSaturationLimit=inf  LowerSaturationLimit=-inf  LinearizeAsGain=on  AntiWindupMode=none  Kb=1  TrackingMode=off  Kt=1  PParamMin=[]  PParamMax=[]  IParamMin=[]  IParamMax=[]  DParamMin=[]  DParamMax=[]  NParamMin=[]  NParamMax=[]  KbParamMin=[]  KbParamMax=[]  KtParamMin=[]  KtParamMax=[]  POutMin=[]  POutMax=[]  IOutMin=[]  IOutMax=[]  DOutMin=[]  DOutMax=[]  NOutMin=[]  NOutMax=[]  KbOutMin=[]  KbOutMax=[]  KtOutMin=[]  KtOutMax=[]  IntegratorOutMin=[]  IntegratorOutMax=[]  FilterOutMin=[]  FilterOutMax=[]  SumOutMin=[]  SumOutMax=[]  SumI1OutMin=[]  SumI1OutMax=[]  SumI2OutMin=[]  SumI2OutMax=[]  SumI3OutMin=[]  SumI3OutMax=[]  SumDOutMin=[]  SumDOutMax=[]  SaturationOutMin=[]  SaturationOutMax=[]  IntegratorContinuousStateAttributes=''  IntegratorStateMustResolveToSignalObject=off  IntegratorRTWStateStorageClass=Auto  FilterContinuousStateAttributes=''  FilterStateMustResolveToSignalObject=off  FilterRTWStateStorageClass=Auto  DifferentiatorICPrevScaledInput=0  DifferentiatorOutMin=[]  DifferentiatorOutMax=[]
  Acceleration Feed : Gain  Gain=KTA(i,i)+(KM(i,i)*KCA(i,i))^-1  Multiplication=Matrix(K*u)
  Constant : Constant  Value=0
  KTA : Gain  Gain=KTA(i,i)  Multiplication=Matrix(K*u)
  KTP : Gain  Gain=KTP(i,i)  Multiplication=Matrix(K*u)
  KTV : Gain  Gain=KTV(i,i)  Multiplication=Matrix(K*u)
  Manual Switch : ManualSwitch  CurrentSetting=0
  Manual Switch1 : ManualSwitch  CurrentSetting=0
  Manual Switch2 : ManualSwitch
  Modello Motore : Subsystem
  Position Controller : simulink/Continuous/PID Controller  Controller=P  TimeDomain=Continuous-time  SampleTime=-1  IntegratorMethod=Forward Euler  FilterMethod=Forward Euler  Form=Parallel  UseFilter=on  ControllerParametersSource=internal  P=KCP(i,i)  I=1  D=0  N=100  InitialConditionSource=internal  InitialConditionForIntegrator=0  InitialConditionForFilter=0  ExternalReset=none  LimitOutput=off  UpperSaturationLimit=inf  LowerSaturationLimit=-inf  LinearizeAsGain=on  AntiWindupMode=none  Kb=1  TrackingMode=off  Kt=1  PParamMin=[]  PParamMax=[]  IParamMin=[]  IParamMax=[]  DParamMin=[]  DParamMax=[]  NParamMin=[]  NParamMax=[]  KbParamMin=[]  KbParamMax=[]  KtParamMin=[]  KtParamMax=[]  POutMin=[]  POutMax=[]  IOutMin=[]  IOutMax=[]  DOutMin=[]  DOutMax=[]  NOutMin=[]  NOutMax=[]  KbOutMin=[]  KbOutMax=[]  KtOutMin=[]  KtOutMax=[]  IntegratorOutMin=[]  IntegratorOutMax=[]  FilterOutMin=[]  FilterOutMax=[]  SumOutMin=[]  SumOutMax=[]  SumI1OutMin=[]  SumI1OutMax=[]  SumI2OutMin=[]  SumI2OutMax=[]  SumI3OutMin=[]  SumI3OutMax=[]  SumDOutMin=[]  SumDOutMax=[]  SaturationOutMin=[]  SaturationOutMax=[]  IntegratorContinuousStateAttributes=''  IntegratorStateMustResolveToSignalObject=off  IntegratorRTWStateStorageClass=Auto  FilterContinuousStateAttributes=''  FilterStateMustResolveToSignalObject=off  FilterRTWStateStorageClass=Auto  DifferentiatorICPrevScaledInput=0  DifferentiatorOutMin=[]  DifferentiatorOutMax=[]
  Position Feed : Gain  Gain=KTP(i,i)  Multiplication=Matrix(K*u)
  Sum : Sum  Inputs=|+-
  Sum1 : Sum  Inputs=++-
  Sum2 : Sum  Inputs=++-
  Velocity Controller : simulink/Continuous/PID Controller  Controller=P  TimeDomain=Continuous-time  SampleTime=-1  IntegratorMethod=Forward Euler  FilterMethod=Forward Euler  Form=Parallel  UseFilter=on  ControllerParametersSource=internal  P=KCV(i,i)  I=1  D=0  N=100  InitialConditionSource=internal  InitialConditionForIntegrator=0  InitialConditionForFilter=0  ExternalReset=none  LimitOutput=off  UpperSaturationLimit=inf  LowerSaturationLimit=-inf  LinearizeAsGain=on  AntiWindupMode=none  Kb=1  TrackingMode=off  Kt=1  PParamMin=[]  PParamMax=[]  IParamMin=[]  IParamMax=[]  DParamMin=[]  DParamMax=[]  NParamMin=[]  NParamMax=[]  KbParamMin=[]  KbParamMax=[]  KtParamMin=[]  KtParamMax=[]  POutMin=[]  POutMax=[]  IOutMin=[]  IOutMax=[]  DOutMin=[]  DOutMax=[]  NOutMin=[]  NOutMax=[]  KbOutMin=[]  KbOutMax=[]  KtOutMin=[]  KtOutMax=[]  IntegratorOutMin=[]  IntegratorOutMax=[]  FilterOutMin=[]  FilterOutMax=[]  SumOutMin=[]  SumOutMax=[]  SumI1OutMin=[]  SumI1OutMax=[]  SumI2OutMin=[]  SumI2OutMax=[]  SumI3OutMin=[]  SumI3OutMax=[]  SumDOutMin=[]  SumDOutMax=[]  SaturationOutMin=[]  SaturationOutMax=[]  IntegratorContinuousStateAttributes=''  IntegratorStateMustResolveToSignalObject=off  IntegratorRTWStateStorageClass=Auto  FilterContinuousStateAttributes=''  FilterStateMustResolveToSignalObject=off  FilterRTWStateStorageClass=Auto  DifferentiatorICPrevScaledInput=0  DifferentiatorOutMin=[]  DifferentiatorOutMax=[]
  Velocity Fedd : Gain  Gain=KTV(i,i)  Multiplication=Matrix(K*u)
  teta : Outport  PortDimensions=1
  dteta : Outport  Port=2  PortDimensions=1
  ddteta : Outport  Port=3  PortDimensions=1
  wires:
  Sum/1 -> Position Controller/1
  Sum1/1 -> Velocity Controller/1
  Sum2/1 -> Acceleration Controller/1
  ddtetad/1 -> Acceleration Feed/1
  KTP/1 -> Sum/2
  Acceleration Controller/1 -> Modello Motore/2(In1)
  dist/1 -> Modello Motore/1(dist)
  Modello Motore/2(dq) -> dteta/1, KTV/1
  Modello Motore/1(q) -> teta/1, KTP/1
  Modello Motore/3(ddq) -> ddteta/1, KTA/1
  Position Controller/1 -> Sum1/2
  KTV/1 -> Sum1/3
  Manual Switch/1 -> Sum1/1
  KTA/1 -> Sum2/3
  Velocity Controller/1 -> Sum2/2
  dtetad/1 -> Velocity Fedd/1
  Constant/1 -> Manual Switch1/2, Manual Switch/2
  Manual Switch1/1 -> Sum2/1
  tetad/1 -> Position Feed/1, Manual Switch2/1
  Manual Switch2/1 -> Sum/1
  Position Feed/1 -> Manual Switch2/2
  Velocity Fedd/1 -> Manual Switch/1
  Acceleration Feed/1 -> Manual Switch1/1
